simulink model "upldl"  (Simulink 4.00)
settings: Solver=FixedStepDiscrete  SolverMode=SingleTasking  StartTime=0.0  StopTime=10.0  FixedStep=0.001  RelTol=1e-3
settings Model: Creator=quaranta  LastModifiedBy=quaranta  SaveTime=off  SaveOutput=off  SimulationMode=external  RTWOptions="-aExtMode=1 -aForceParamTrailComments=0 -aInlineInvariantSignals=0 -aLocalBlockOutputs=1 -aLogVarNameModifier=\"rt_\" -aRTWVerbose=1 -aRollThreshold=5 -aShowEliminatedStatements=1"  RTWTemplateMakefile=grt_rtai.tmf  ExtModeTrigDuration=10000  BlockReductionOpt=off

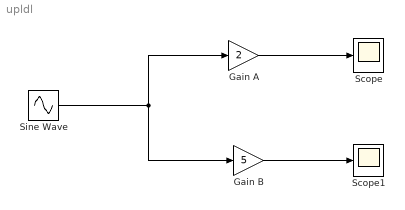
== system upldl ==
  Gain A : Gain  Gain=2  Multiplication=Element-wise(K.*u)  SaturateOnIntegerOverflow=on
  Gain B : Gain  Gain=5  Multiplication=Element-wise(K.*u)  SaturateOnIntegerOverflow=on
  Scope : Scope
      settings: TimeRange=3  YMin=-5  YMax=5  SaveToWorkspace=off  SaveName=ScopeData  MaxDataPoints=5000
  Scope1 : Scope
      settings: TimeRange=auto  YMin=-5  YMax=5  SaveToWorkspace=off  LimitDataPoints=on  MaxDataPoints=5000
  Sine Wave : Sin  Amplitude=1  Frequency=1  Phase=0  SampleTime=0
  wires:
  Sine Wave/1 -> Gain A/1, Gain B/1
  Gain A/1 -> Scope/1
  Gain B/1 -> Scope1/1
